simulink model "DK_hoi_tiep_tuyen_tinh_hoa"  (R2023a)
settings: Solver=ode4  StartTime=0.0  StopTime=50  FixedStep=0.001  RelTol=1e-3
settings Model: Creator=VINH  LastModifiedBy=VINH

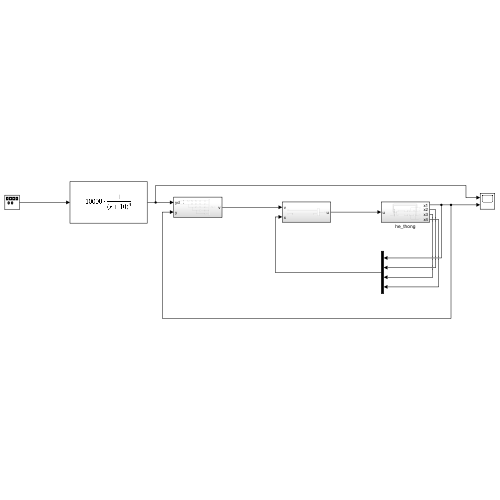
[thumbnail: Simulink's stored preview of the top-level diagram]
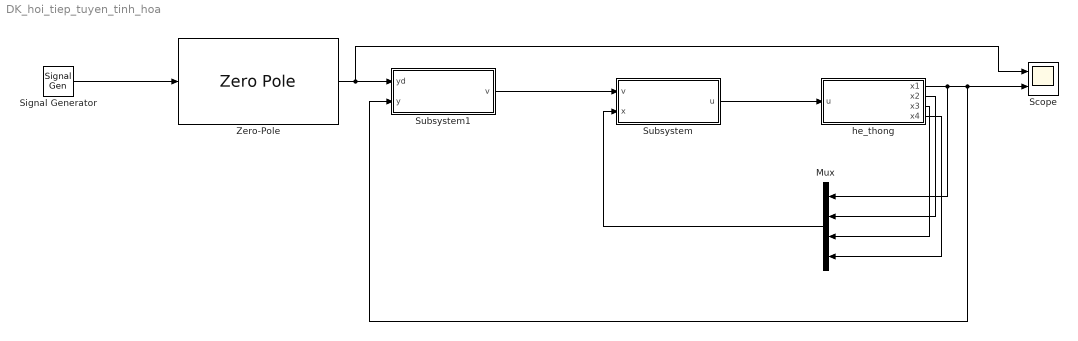
== system DK_hoi_tiep_tuyen_tinh_hoa ==
  Mux : Mux
  Scope : Scope  NumInputPorts=2
  Signal Generator : SignalGenerator  WaveForm=square  Amplitude=0.5  Frequency=0.1
  Subsystem : Subsystem
  Subsystem1 : Subsystem
  Zero-Pole : ZeroPole  Zeros=[]  Poles=[-10 -10 -10 -10]  Gain=10000
  he_thong : Subsystem
  wires:
  Subsystem/1(u) -> he_thong/1(u)
  he_thong/1(x1) -> Mux/1, Scope/2, Subsystem1/2(y)
  he_thong/2(x2) -> Mux/2
  he_thong/3(x3) -> Mux/3
  he_thong/4(x4) -> Mux/4
  Mux/1 -> Subsystem/2(x)
  Subsystem1/1(v) -> Subsystem/1(v)
  Signal Generator/1 -> Zero-Pole/1
  Zero-Pole/1 -> Subsystem1/1(yd), Scope/1

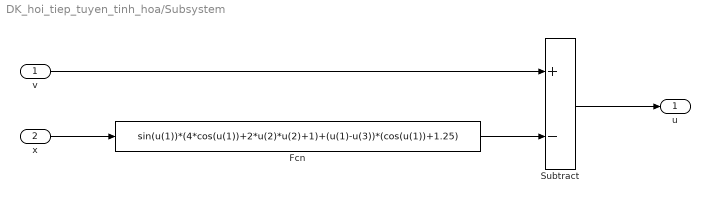
== system DK_hoi_tiep_tuyen_tinh_hoa/Subsystem ==
  v : Inport
  x : Inport  Port=2
  Fcn : Fcn  Expr=sin(u(1))*(4*cos(u(1))+2*u(2)*u(2)+1)+(u(1)-u(3))*(cos(u(1))+1.25)
  Subtract : Sum  Inputs=+-
  u : Outport
  wires:
  v/1 -> Subtract/1
  x/1 -> Fcn/1
  Fcn/1 -> Subtract/2
  Subtract/1 -> u/1

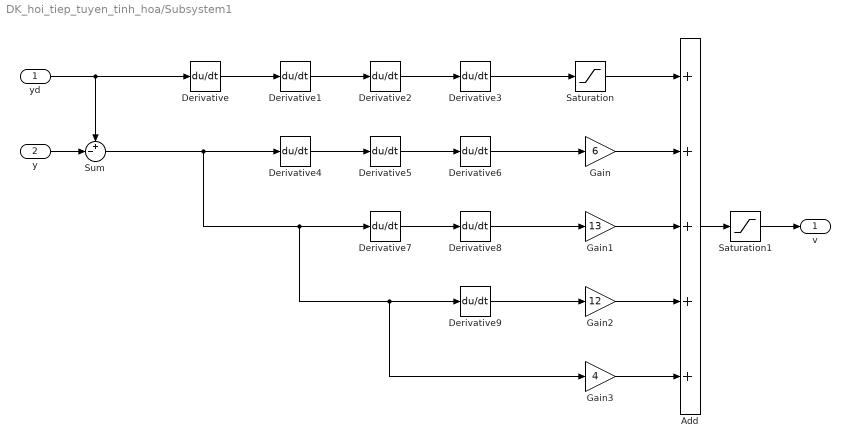
== system DK_hoi_tiep_tuyen_tinh_hoa/Subsystem1 ==
  yd : Inport
  y : Inport  Port=2
  Add : Sum  Inputs=+++++
  Derivative{,1..9} (10 alike) : Derivative
  Gain : Gain  Gain=6
  Gain1 : Gain  Gain=13
  Gain2 : Gain  Gain=12
  Gain3 : Gain  Gain=4
  Saturation : Saturate  UpperLimit=2  LowerLimit=-2
  Saturation1 : Saturate  UpperLimit=5  LowerLimit=-5
  Sum : Sum  Inputs=+-|
  v : Outport
  wires:
  yd/1 -> Derivative/1, Sum/1
  y/1 -> Sum/2
  Derivative/1 -> Derivative1/1
  Derivative1/1 -> Derivative2/1
  Derivative2/1 -> Derivative3/1
  Sum/1 -> Derivative4/1, Derivative7/1, Derivative9/1, Gain3/1
  Derivative4/1 -> Derivative5/1
  Derivative5/1 -> Derivative6/1
  Derivative7/1 -> Derivative8/1
  Derivative6/1 -> Gain/1
  Derivative8/1 -> Gain1/1
  Derivative9/1 -> Gain2/1
  Gain/1 -> Add/2
  Gain1/1 -> Add/3
  Gain2/1 -> Add/4
  Add/1 -> Saturation1/1
  Gain3/1 -> Add/5
  Derivative3/1 -> Saturation/1
  Saturation1/1 -> v/1
  Saturation/1 -> Add/1

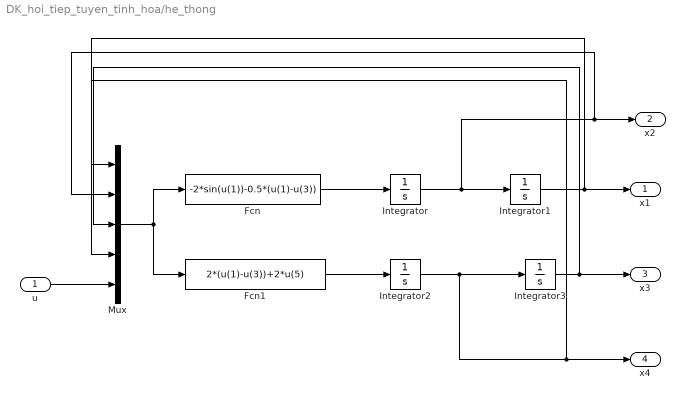
== system DK_hoi_tiep_tuyen_tinh_hoa/he_thong ==
  u : Inport
  Fcn : Fcn  Expr=-2*sin(u(1))-0.5*(u(1)-u(3))
  Fcn1 : Fcn  Expr=2*(u(1)-u(3))+2*u(5)
  Integrator{,1..3} (4 alike) : Integrator
  Mux : Mux  Inputs=5
  x1 : Outport
  x2 : Outport  Port=2
  x3 : Outport  Port=3
  x4 : Outport  Port=4
  wires:
  Integrator/1 -> Mux/2, x2/1, Integrator1/1
  Integrator2/1 -> x4/1, Mux/4, Integrator3/1
  Mux/1 -> Fcn1/1, Fcn/1
  Fcn/1 -> Integrator/1
  Integrator1/1 -> Mux/1, x1/1
  Fcn1/1 -> Integrator2/1
  Integrator3/1 -> Mux/3, x3/1
  u/1 -> Mux/5
